simulink model "SG_GFOL_2020a"  (R2024a)
settings: Solver=ode1  StartTime=0.0  StopTime=Tsim  FixedStep=Ts  MaxStep=1e-4  RelTol=1e-4  EnableMultiTasking=on
values from neighbouring files (symbols this model uses):
  f1 = 50    [VSC_GF_SG_params.m]
  H = 5    [VSC_GF_SG_params.m]
  Inom_n2 = Sn_n2/Un_n2/sqrt(3)    [VSC_GF_SG_params.m]
  k_droop_f_n2 = 1/0.05    (= 20)    [VSC_GF_SG_params.m]
  ki_p_n2 = 1/tau_p    (= 5)    [VSC_GF_SG_params.m]
  ki_pll1 = kp_pll1/tau_pll_n1    [VSC_GF_SG_params.m]
  ki_pll_n2 = kp_pll_n2/tau_pll_n2    [VSC_GF_SG_params.m]
  ki_q_n2 = 1/tau_q    (= 5)    [VSC_GF_SG_params.m]
  ki_s_n2 = Rc_n2/taus_n2    (= 2048)    [VSC_GF_SG_params.m]
  kp_p_n2 = taus_n2/tau_p    (= 0.005)    [VSC_GF_SG_params.m]
  kp_pll1 = xi_pll_n1*2*omega_pll_n1/Vpeak    [VSC_GF_SG_params.m]
  kp_pll_n2 = xi_pll_n2*2*omega_pll_n2/Vpeak_n2    [VSC_GF_SG_params.m]
  kp_q_n2 = taus_n2/tau_q    (= 0.005)    [VSC_GF_SG_params.m]
  kp_s_n2 = Lc_n2/taus_n2    (= 130.379729381)    [VSC_GF_SG_params.m]
  Lac = Lpu*l*(Un1/Vl)^2    (= 0.105785123967)    [VSC_GF_SG_params.m]
  Lc_n2 = 0.2*Ln_n2    (= 0.130379729381)    [VSC_GF_SG_params.m]
  magnitud_delay = Ts    (= 5e-05)    [VSC_GF_SG_params.m]
  Pload_fnl = 400e6    (= 400000000)    [VSC_GF_SG_params.m]
  plots_step = Ts    (= 5e-05)    [VSC_GF_SG_params.m]
  Psg0_pu = Psg0/Pn    (= 0.4)    [VSC_GF_SG_params.m]
  Pvsc0 = Pload0 -Psg0    (= 200000000)    [VSC_GF_SG_params.m]
  Q_ref_n2 = 0e6    (= 0)    [VSC_GF_SG_params.m]
  Rac = Rpu*l*(Un1/Vl)^2    (= 3.17355371901)    [VSC_GF_SG_params.m]
  Rc_n2 = 0.01*Xn_n2    (= 2.048)    [VSC_GF_SG_params.m]
  Sn_n2 = Sn1    (= 500000000)    [VSC_GF_SG_params.m]
  Ssg = 500e6    (= 500000000)    [VSC_GF_SG_params.m]
  T_stp = 20    [VSC_GF_SG_params.m]
  tau_droop_fpll = 0.1    [VSC_GF_SG_params.m]
  tau_u = 40e-3    (= 0.04)    [VSC_GF_SG_params.m]
  Ts = 5e-5    (= 5e-05)    [VSC_GF_SG_params.m]
  Tsim = 40    [VSC_GF_SG_params.m]
  Un1 = 320e3    (= 320000)    [VSC_GF_SG_params.m]
  Vdcref_n1 = 640e3    (= 640000)    [VSC_GF_SG_params.m]
  Vpeak = Un1*sqrt(2/3)    [VSC_GF_SG_params.m]
  Vpeak_n1 = Un_n1/sqrt(3)*sqrt(2)    [VSC_GF_SG_params.m]
  Vpeak_n2 = Un_n2/sqrt(3)*sqrt(2)    [VSC_GF_SG_params.m]
  w_g1 = 2*pi*f1    (= 314.159265359)    [VSC_GF_SG_params.m]
  w_n2 = 2*pi*f_n2    (= 314.159265359)    [VSC_GF_SG_params.m]
undefined symbols (not defined in the file or in its folder): D11, Delta, k, magnitude, P_set, P_step, Pload_init, Q_set, Q_step, t_ramp, t_step_P, t_step_Q, tau_ramp, tau_wf
libraries: simulink x6, simulink_extras x6, spsSeriesRLCBranchLib x6, spsThreePhaseParallelRLCLoadLib x4, spsControlledVoltageSourceLib x4, spsCurrentMeasurementLib x4, spsControlledCurrentSourceLib x3, spsVoltageMeasurementLib x3, spsLoadFlowBusLib x2, slpidlib x2, spsGroundLib x2, spsSampleandHoldLib x1
(part 1 of 2)
settings Model: ExtModeTrigDuration=100  Creator=Enric  LastModifiedBy=citcea
settings SolverCC: SolverJacobianMethodControl=FullPerturbation  AlgebraicLoopSolver=TrustRegion
settings DataIOCC: LimitDataPoints=on  SaveOutput=off  ReturnWorkspaceOutputs=off  StateSaveName=tmp_raccel_xout  SignalLoggingName=tmp_raccel_logsout
settings OptimizationCC: EfficientMapNaN2IntZero=off  LifeSpan=inf
settings DebuggingCC: UnconnectedInputMsg=warning  UnconnectedOutputMsg=warning  UnconnectedLineMsg=warning  AllowSymbolicDim=off  SFUnexpectedBacktrackingDiag=warning  SFNoUnconditionalDefaultTransitionDiag=warning  SFExecutionAtInitializationDiag=none  ArithmeticOperatorsInVariantConditions=warning
settings HardwareCC: TargetBitPerPointer=64  TargetBitPerSizeT=64  TargetBitPerPtrDiffT=64  TargetLongLongMode=on  TargetIntDivRoundTo=Zero  TargetEndianess=LittleEndian  TargetWordSize=64  TargetHWDeviceType=MATLAB Host  ProdEqTarget=off
settings ModelReferenceCC: EnableRefExpFcnMdlSchedulingChecks=on  PropagateSignalLabelsOutOfModel=off
settings SFSimCC: SimUseLocalCustomCode=off  CustomCodeUndefinedFunction=UseInterfaceOnly
settings RTWCC: SystemTargetFile=raccel.tlc  TemplateMakefile=raccel_default_tmf  RTWVerbose=off  RTWUseLocalCustomCode=off  RTWUseSimCustomCode=on  GPUComputeCapability=3.5
settings CodeAppCC: GenerateComments=off  MaxIdLength=128  MangleLength=10  SimulinkBlockComments=off
settings RaccelTargetCC: InstructionSetFMA=off  OptimizeReductions=off  LogToMDFFile=off  ENABLE_SLEXEC_SSBRIDGE=0  RTWCAPISignals=off  RTWCAPIParams=on  RTWCAPIRootIO=off
settings ConfigComp: CovMetricSettings=dw  CovSaveCumulativeToWorkspaceVar=on  CovSaveSingleToWorkspaceVar=on  CovExternalEMLEnable=off
settings SimscapeCC: SimscapeNormalizeSystem=off

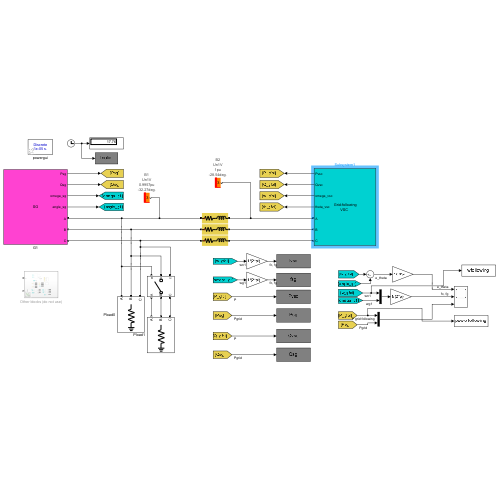
[thumbnail: Simulink's stored preview of the top-level diagram]
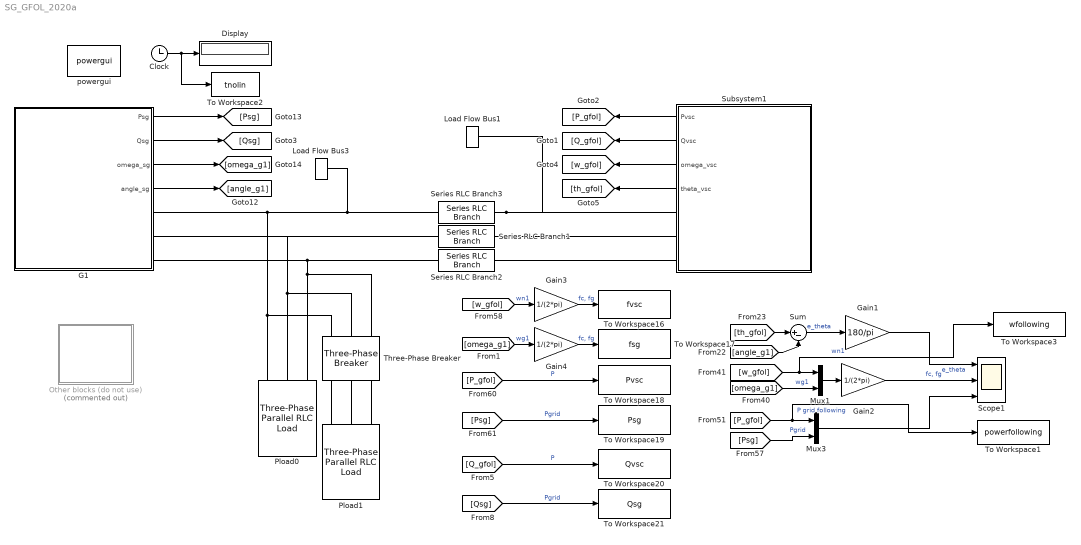
== system SG_GFOL_2020a ==
  Clock : Clock
  Display : Display
  G1 : Subsystem
      mask Display:
      | disp('SG')
      | %x = [0:0.001:1];
      | %y = 0.2*sin(10*x) + 0.5;
      | %plot(x,y)
  Gain1 : Gain  Gain=180/pi
  Gain2 : Gain  Gain=1/(2*pi)
  Gain3 : Gain  Gain=1/(2*pi)
  Gain4 : Gain  Gain=1/(2*pi)
  Load Flow Bus1 : spsLoadFlowBusLib/Load Flow Bus  LConnTagsString=a  Phases=single  Connectors=on one side  ID=B2  Vbase=Un1  Vref=1  Vangle=0  VLF=1  VLFb=1  VLFc=1  angleLF=-28.54  angleLFb=0  angleLFc=0
  Load Flow Bus3 : spsLoadFlowBusLib/Load Flow Bus  LConnTagsString=a  Phases=single  Connectors=on one side  ID=B1  Vbase=Un1  Vref=1  Vangle=0  VLF=0.9957  VLFb=1  VLFc=1  angleLF=-32.27  angleLFb=0  angleLFc=0
  Mux1 : Mux  Inputs=2
  Mux3 : Mux  Inputs=2
  Other blocks (do not use) : Subsystem  Commented=on
  Pload0 : spsThreePhaseParallelRLCLoadLib/Three-Phase Parallel RLC Load  LConnTagsString=A|B|C  Configuration=Y (grounded)  NominalVoltage=Vsg  Vabc=[1e3 1e3 1e3]  Vabcp=[1e3 1e3 1e3]  NominalFrequency=50  UnbalancedPower=off  ActivePower=Pload0  InductivePower=0  CapacitivePower=0  Pabc=[10e3 9e3 11e3]  QLabc=[100 90 110]  QCabc=[100 90 110]  Pabcp=[10e3 9e3 11e3]  QLabcp=[100 90 110]  QCabcp=[100 90 110]  Measurements=None  LoadType=constant Z
  Pload1 : spsThreePhaseParallelRLCLoadLib/Three-Phase Parallel RLC Load  LConnTagsString=A|B|C  Configuration=Y (grounded)  NominalVoltage=Vsg  Vabc=[1e3 1e3 1e3]  Vabcp=[1e3 1e3 1e3]  NominalFrequency=50  UnbalancedPower=off  ActivePower=Pload1  InductivePower=0  CapacitivePower=0  Pabc=[10e3 9e3 11e3]  QLabc=[100 90 110]  QCabc=[100 90 110]  Pabcp=[10e3 9e3 11e3]  QLabcp=[100 90 110]  QCabcp=[100 90 110]  Measurements=None  LoadType=constant Z
  Scope1 : Scope  NumInputPorts=3
  Series RLC Branch1 : spsSeriesRLCBranchLib/Series RLC Branch  LConnTagsString=__new0  RConnTagsString=__new0  BranchType=RL  Resistance=Rac  Inductance=Lac  SetiL0=off  InitialCurrent=0  Capacitance=0  Setx0=off  InitialVoltage=0  Measurements=None
  Series RLC Branch2 : spsSeriesRLCBranchLib/Series RLC Branch  LConnTagsString=__new0  RConnTagsString=__new0  BranchType=RL  Resistance=Rac  Inductance=Lac  SetiL0=off  InitialCurrent=0  Capacitance=0  Setx0=off  InitialVoltage=0  Measurements=None
  Series RLC Branch3 : spsSeriesRLCBranchLib/Series RLC Branch  LConnTagsString=__new0  RConnTagsString=__new0  BranchType=RL  Resistance=Rac  Inductance=Lac  SetiL0=off  InitialCurrent=0  Capacitance=0  Setx0=off  InitialVoltage=0  Measurements=None
  Subsystem1 : Subsystem
      mask Display: disp('VSC \n Grid-following')
  Sum : Sum  Inputs=|+-
  Three-Phase Breaker : spsThreePhaseBreakerLib/Three-Phase Breaker  InitialState=open  SwitchA=on  SwitchB=on  SwitchC=on  SwitchTimes=[T_stp 1000]  External=off  BreakerResistance=0.0001  SnubberResistance=inf  SnubberCapacitance=inf  Measurements=None
  To Workspace1 : ToWorkspace  VariableName=powerfollowing  SaveFormat=Timeseries  SampleTime=-1
  To Workspace16 : ToWorkspace  VariableName=fvsc  SampleTime=plots_step
  To Workspace17 : ToWorkspace  VariableName=fsg  SampleTime=plots_step
  To Workspace18 : ToWorkspace  VariableName=Pvsc  SampleTime=plots_step
  To Workspace19 : ToWorkspace  VariableName=Psg  SampleTime=plots_step
  To Workspace2 : ToWorkspace  VariableName=tnolin  SampleTime=plots_step
  To Workspace20 : ToWorkspace  VariableName=Qvsc  SampleTime=plots_step
  To Workspace21 : ToWorkspace  VariableName=Qsg  SampleTime=plots_step
  To Workspace3 : ToWorkspace  VariableName=wfollowing  SaveFormat=Timeseries  SampleTime=-1
  powergui : sps_lib/powergui  Priority=1  SimulationMode=Discrete  SampleTime=Ts  frequency=50  Iterations=50  frequencyindice=0  Pbase=100e6  ErrMax=0.0001  UnitsV=kV  UnitsW=MW  buscounter=0  FunctionMessages=off  echomessages=off  EnableUseOfTLC=off  CurrentSourceSwitches=off  DisableSnubberDevices=off  DisableRonSwitches=off  DisableVfSwitches=off  DisplayEquations=off  AutomaticDiscreteSolvers=off  SolverType=Tustin  Interpol=off  ExternalGateDelay=off  methode=off  Ts=0  x0status=blocks  SPID=off  SwTol=0  HookPort=off  NonlinearTolerance=1e-4  nMaxIteration=100  ContinueOnMaxIteration=off  RestoreLinks=warning  ResistiveCurrentMeasurement=off  Frange=[0:2:500]  Ylog=off  Xlog=on  ShowGrid=off  save=off  variable=ZData  structure=Vk  ZoomFFT=off  StartTime=2.01  cycles=3  DisplayStyle=1  fundamental=50  FreqAxis=off  MaxFrequency=1000  frequencyindicesteady=1  RmsSteady=1  display=off
  wires:
  Clock/1 -> To Workspace2/1, Display/1
  [th_gfol] -> Sum/1
  [angle_g1] -> Sum/2
  Sum/1 -> Gain1/1  "e_theta"
  [w_gfol] -> To Workspace3/1, Mux1/1  "wn1"
  [omega_g1] -> Mux1/2  "wg1"
  Mux1/1 -> Gain2/1
  Gain2/1 -> Scope1/2  "fc, fg"
  Gain1/1 -> Scope1/1  "e_theta"
  [P_gfol] -> To Workspace1/1, Mux3/1  "P grid following"
  [Psg] -> Mux3/2  "Pgrid"
  Mux3/1 -> Scope1/3
  [w_gfol] -> Gain3/1  "wn1"
  Gain3/1 -> To Workspace16/1  "fc, fg"
  Gain4/1 -> To Workspace17/1  "fc, fg"
  [omega_g1] -> Gain4/1  "wg1"
  [P_gfol] -> To Workspace18/1  "P"
  [Psg] -> To Workspace19/1  "Pgrid"
  G1/1(Psg) -> [Psg]
  G1/3(omega_sg) -> [omega_g1]
  G1/4(angle_sg) -> [angle_g1]
  Subsystem1/4(theta_vsc) -> [th_gfol]
  Subsystem1/3(omega_vsc) -> [w_gfol]
  Subsystem1/1(Pvsc) -> [P_gfol]
  Subsystem1/2(Qvsc) -> [Q_gfol]
  [Qsg] -> To Workspace21/1  "Pgrid"
  [Q_gfol] -> To Workspace20/1  "P"
  G1/2(Qsg) -> [Qsg]
  connections:
  Series RLC Branch1/LConn1 -- G1/RConn2 -- Three-Phase Breaker/RConn2 -- Pload0/LConn2
  Series RLC Branch3/RConn1 -- Subsystem1/RConn1 -- Load Flow Bus1/LConn1
  Subsystem1/RConn2 -- Series RLC Branch1/RConn1
  Subsystem1/RConn3 -- Series RLC Branch2/RConn1
  Load Flow Bus3/LConn1 -- Series RLC Branch3/LConn1 -- Three-Phase Breaker/RConn1 -- Pload0/LConn1 -- G1/RConn1
  Three-Phase Breaker/LConn1 -- Pload1/LConn1
  Pload1/LConn2 -- Three-Phase Breaker/LConn2
  Three-Phase Breaker/LConn3 -- Pload1/LConn3
  Series RLC Branch2/LConn1 -- Three-Phase Breaker/RConn3 -- Pload0/LConn3 -- G1/RConn3

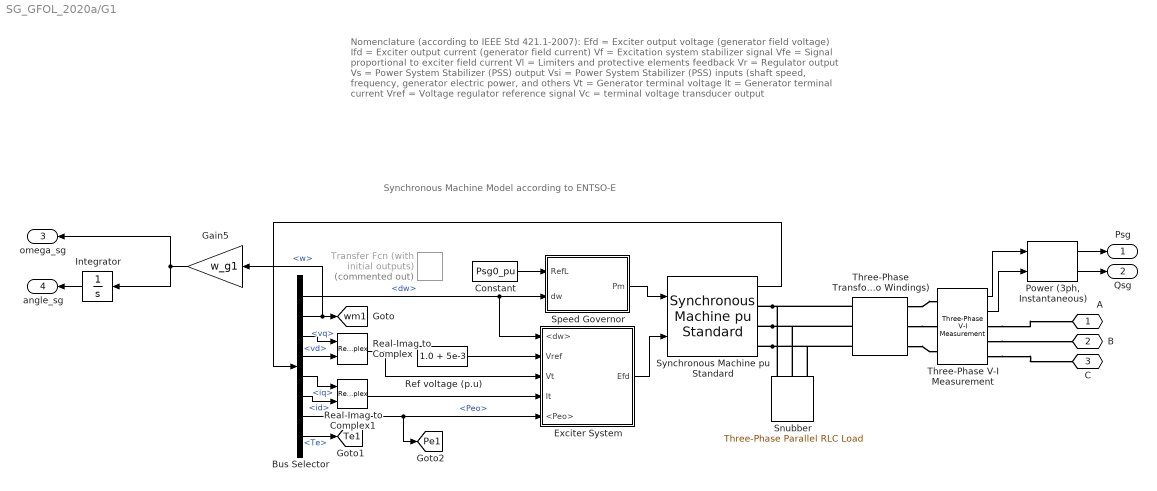
== system SG_GFOL_2020a/G1 ==
  note: Synchronous Machine Model according to ENTSO-E
  note: Nomenclature (according to IEEE Std 421.1-2007):
      | Efd = Exciter output voltage (generator field voltage)
      | Ifd = Exciter output current (generator field current)
      | Vf = Excitation system stabilizer signal
      | Vfe = Signal proportional to exciter field current
      | Vl = Limiters and protective elements feedback
      | Vr = Regulator output
      | Vs = Power System Stabilizer (PSS) output
      | Vsi = Power System Stabilizer (PSS) inputs (shaft speed, frequency, generator electric power, and others
      | Vt = Generator terminal voltage
      | It = Generator terminal current
      | Vref = Voltage regulator reference signal
      | Vc = terminal voltage transducer output
  Bus Selector : BusSelector  OutputSignals=dw,w,vq,vd,iq,id,Peo,Te
  Constant : Constant  Value=Psg0_pu
  Exciter System : Subsystem
  Gain5 : Gain  Gain=w_g1
  Integrator : Integrator
  "Power (3ph, Instantaneous)" : spsPower3phInstantaneousLib/Power (3ph, Instantaneous)
  Real-Imag to Complex : RealImagToComplex
  Real-Imag to Complex1 : RealImagToComplex
  Ref voltage (p.u) : Constant  Value=1.0 + 5e-3
  Snubber : spsThreePhaseParallelRLCLoadLib/Three-Phase Parallel RLC Load  LConnTagsString=A|B|C  Configuration=Y (grounded)  NominalVoltage=Un1  Vabc=[1e3 1e3 1e3]  Vabcp=[1e3 1e3 1e3]  NominalFrequency=f1  UnbalancedPower=off  ActivePower=Ssg*0.01  InductivePower=0  CapacitivePower=0  Pabc=[10e3 9e3 11e3]  QLabc=[100 90 110]  QCabc=[100 90 110]  Pabcp=[10e3 9e3 11e3]  QLabcp=[100 90 110]  QCabcp=[100 90 110]  Measurements=None  LoadType=constant Z
  Speed Governor : Subsystem  mask{R=0.05, T1=0.5, T2=3, T3=10, Dt=0, Vmin=0, Vmax=10, P0=Psg0_pu}
      mask prompts: R "Controller droop (R)"; T1 "Governor time constant (T1)(sec)"; T2 "Turbine derivative time constant (T2)(sec)"; T3 "Turbine delay time constant (T3)(sec)"; Dt "Frictional losses factor (Dt)"; Vmin "Minimum gate limit (Vmin)(p.u)"; Vmax "Maximum gate limit (Vmax)(p.u)"; P0 "Initial power (p.u)"
      mask Display:
      | disp('TGOV')
      | 
      | port_label('input',1,'Pref')
      | port_label('input',2,'dw')
      | 
      | port_label('output',1,'Pm')
  Synchronous Machine pu Standard : spsSynchronousMachinepuStandardLib/Synchronous Machine pu Standard  PresetModel=No  MechanicalLoad=Mechanical power Pm  ShowDetailedParameters=on  RotorType=Salient-pole  Units=per unit standard parameters  MeasurementBus=on  NominalParameters=[Ssg Un1 f1]  Reactances1=[ 1.81, 0.3, 0.23, 1.76, 0.65, 0.25, 0.15 ]  Reactances2=[1.25 0.333 0.292 1.0 0.292 0.15]  dAxisTimeConstants=Open-circuit  qAxisTimeConstants=Open-circuit  TimeConstants1="[5  0.002  0.002]"  TimeConstants2=[ 8.0, 0.03, 1.0, 0.07 ]  TimeConstants3="[  4.49  0.0681  0.0513  ]"  TimeConstants4=[ 8.0, 0.03, 0.3371, 0.0295 ]  TimeConstants5=[ 1.01, 0.053, 0.1 ]  TimeConstants6=[ 1.3201, 0.023, 1.0, 0.07 ]  TimeConstants7=[0.012 0.003 0.003]  TimeConstants8=[ 1.3201, 0.0231, 0.3371, 0.0295 ]  StatorResistance=0.01  Mechanical=[H 0 2]  PolePairs=20  InitialConditions=[0 -68.7735 0.408291 0.408291 0.408291 -5.73726 -125.737 114.263 1.16721]  SetSaturation=off  Saturation=[0.6404,0.7127,0.8441,0.9214,0.9956,1.082,1.19,1.316,1.457;0.7,0.7698,0.8872,0.9466,0.9969,1.046,1.1,1.151,1.201]  LoadFlowParameters=[1,0,0,0,0]  TsPowergui=0  TsBlock=-1  IterativeModel=Trapezoidal non iterative  IterativeDiscreteModel=Trapezoidal non iterative  BusType=swing  Pref=0  Qref=0  Qmin=-inf  Qmax=inf  PLF=0  QLF=0
  Three-Phase Transformer (Two Windings) : spsThreePhaseTransformerTwoWindingsLib/Three-Phase Transformer (Two Windings)  Winding1Connection=Delta (D11)  Winding2Connection=Yg  CoreType=Three single-phase transformers  SetSaturation=off  Hysteresis=off  DataFile='hysteresis'  SetInitialFlux=off  Measurements=None  UNITS=pu  NominalPower=[Ssg , f1 ]  Winding1=[Un1 0.00125 0.05]  Winding2=[Un1 0.00125 0.05]  Rm=5000  Lm=5000  L0=0.5  Saturation=[ 0,0 ; 0.0024,1.2 ; 1.0,1.52 ]  InitialFluxes=[ 0.8 , -0.8 , 0.7 ]  BreakLoop=off  DiscreteSolver=Trapezoidal iterative  DataType=off  TransfoNumber=1
  Three-Phase V-I Measurement : spsThreePhaseVIMeasurementLib/Three-Phase V-I Measurement  VoltageMeasurement=phase-to-ground  SetLabelV=off  LabelV=Vabc  Vpu=off  VpuLL=off  CurrentMeasurement=yes  SetLabelI=off  LabelI=Iabc  Ipu=off  Pbase=100e6  Vbase=500e3  OutputType=Complex  PhasorSimulation=off  PSBequivalent=0
  Transfer Fcn (with initial outputs) : simulink_extras/Additional Linear/Transfer Fcn (with initial outputs)  Commented=on  N=[-1.8]  D="[1  0]"  Y0=0.0705  U0=0
  A : PMIOPort  Side=Right
  B : PMIOPort  Port=2  Side=Right
  C : PMIOPort  Port=3  Side=Right
  Psg : Outport
  Qsg : Outport  Port=2
  omega_sg : Outport  Port=3
  angle_sg : Outport  Port=4
  tag scope: Pe1=global, Te1=global, wm1=global
  wires:
  Ref voltage (p.u)/1 -> Exciter System/2(Vref)
  Bus Selector/1 -> Exciter System/1(<dw>), Speed Governor/2(dw)  "<dw>"
  Bus Selector/4 -> Real-Imag to Complex/2  "<vd>"
  Bus Selector/3 -> Real-Imag to Complex/1  "<vq>"
  Bus Selector/5 -> Real-Imag to Complex1/1  "<iq>"
  Bus Selector/6 -> Real-Imag to Complex1/2  "<id>"
  Real-Imag to Complex/1 -> Exciter System/3(Vt)
  Real-Imag to Complex1/1 -> Exciter System/4(It)
  Bus Selector/7 -> Exciter System/5(<Peo>), [Pe1]  "<Peo>"
  Bus Selector/8 -> [Te1]  "<Te>"
  Speed Governor/1(Pm) -> Synchronous Machine pu Standard/1
  Exciter System/1(Efd) -> Synchronous Machine pu Standard/2
  Synchronous Machine pu Standard/1 -> Bus Selector/1
  Constant/1 -> Speed Governor/1(RefL)
  Bus Selector/2 -> Gain5/1, [wm1]  "<w>"
  Integrator/1 -> angle_sg/1
  Gain5/1 -> Integrator/1, omega_sg/1
  Three-Phase V-I Measurement/2 -> "Power (3ph, Instantaneous)"/2
  Three-Phase V-I Measurement/1 -> "Power (3ph, Instantaneous)"/1
  "Power (3ph, Instantaneous)"/1 -> Psg/1
  "Power (3ph, Instantaneous)"/2 -> Qsg/1
  connections:
  Synchronous Machine pu Standard/RConn1 -- Three-Phase Transformer (Two Windings)/LConn1 -- Snubber/LConn1
  Synchronous Machine pu Standard/RConn3 -- Three-Phase Transformer (Two Windings)/LConn3 -- Snubber/LConn3
  Synchronous Machine pu Standard/RConn2 -- Three-Phase Transformer (Two Windings)/LConn2 -- Snubber/LConn2
  Three-Phase Transformer (Two Windings)/RConn2 -- Three-Phase V-I Measurement/LConn2
  Three-Phase Transformer (Two Windings)/RConn1 -- Three-Phase V-I Measurement/LConn1
  Three-Phase Transformer (Two Windings)/RConn3 -- Three-Phase V-I Measurement/LConn3
  Three-Phase V-I Measurement/RConn1 -- A/RConn1
  Three-Phase V-I Measurement/RConn2 -- B/RConn1
  Three-Phase V-I Measurement/RConn3 -- C/RConn1

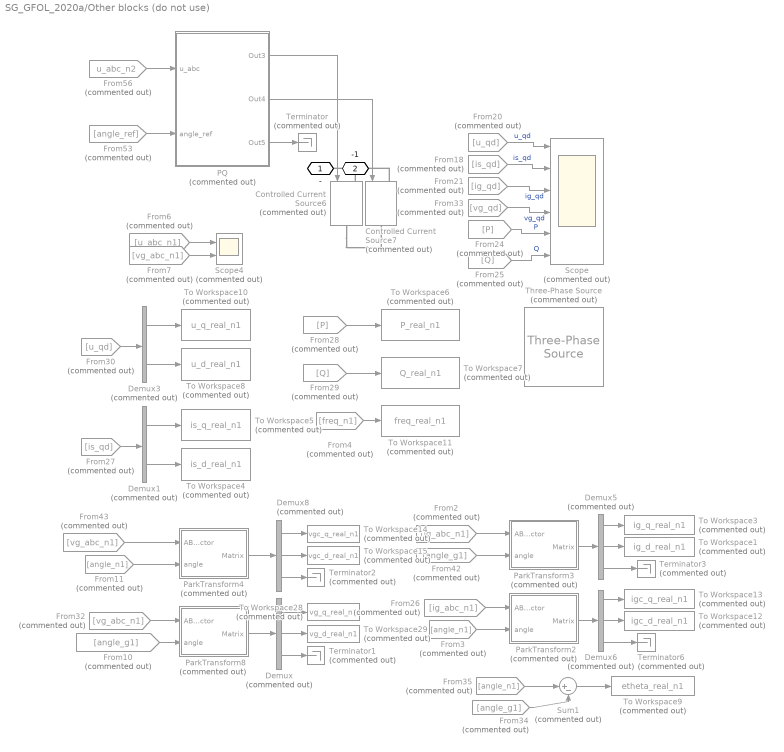
== system SG_GFOL_2020a/Other blocks (do not use) ==
  Controlled Current Source6 : spsControlledCurrentSourceLib/Controlled Current Source  Commented=on  Initialize=off  Source_Type=AC  Amplitude=0  Phase=0  Frequency=0  Measurements=None
  Controlled Current Source7 : spsControlledCurrentSourceLib/Controlled Current Source  Commented=on  Initialize=off  Source_Type=AC  Amplitude=0  Phase=0  Frequency=0  Measurements=None
  Demux{,5..6,8} (4 alike) : Demux  Commented=on  Outputs=3
  Demux1 : Demux  Commented=on  Outputs=2
  Demux3 : Demux  Commented=on  Outputs=2
  From10 : From  Commented=on  GotoTag=angle_g1
  From11 : From  Commented=on  GotoTag=angle_n1
  From18 : From  Commented=on  GotoTag=is_qd
  From2 : From  Commented=on  GotoTag=ig_abc_n1
  From20 : From  Commented=on  GotoTag=u_qd
  From21 : From  Commented=on  GotoTag=ig_qd
  From24 : From  Commented=on  GotoTag=P
  From25 : From  Commented=on  GotoTag=Q
  From26 : From  Commented=on  GotoTag=ig_abc_n1
  From27 : From  Commented=on  GotoTag=is_qd
  From28 : From  Commented=on  GotoTag=P
  From29 : From  Commented=on  GotoTag=Q
  From3 : From  Commented=on  GotoTag=angle_n1
  From30 : From  Commented=on  GotoTag=u_qd
  From32 : From  Commented=on  GotoTag=vg_abc_n1
  From33 : From  Commented=on  GotoTag=vg_qd
  From34 : From  Commented=on  GotoTag=angle_g1
  From35 : From  Commented=on  GotoTag=angle_n1
  From4 : From  Commented=on  GotoTag=freq_n1
  From42 : From  Commented=on  GotoTag=angle_g1
  From43 : From  Commented=on  GotoTag=vg_abc_n1
  From53 : From  Commented=on  GotoTag=angle_ref
  From56 : From  Commented=on  GotoTag=u_abc_n2  TagVisibility=global
  From6 : From  Commented=on  GotoTag=u_abc_n1
  From7 : From  Commented=on  GotoTag=vg_abc_n1
  PQ : Subsystem  Commented=on
  ParkTransform2 : Subsystem  Commented=on  mask(Gerard){}
      mask help:
      | This block applies the park transfomation from a desired vector.
      | The input Xabc refers to the vector in the ABC frame, and the second input is the angle used in the transformation.
      | The output is the vector in the qd0 frame.
      mask Display:
      | port_label('output',1,'Xqd0')
      | port_label('input',1,'Xabc')
      | port_label('input',2,'angle')
  ParkTransform3 : Subsystem  Commented=on  mask(Gerard){}
      mask help:
      | This block applies the park transfomation from a desired vector.
      | The input Xabc refers to the vector in the ABC frame, and the second input is the angle used in the transformation.
      | The output is the vector in the qd0 frame.
      mask Display:
      | port_label('output',1,'Xqd0')
      | port_label('input',1,'Xabc')
      | port_label('input',2,'angle')
  ParkTransform4 : Subsystem  Commented=on  mask(Gerard){}
      mask help:
      | This block applies the park transfomation from a desired vector.
      | The input Xabc refers to the vector in the ABC frame, and the second input is the angle used in the transformation.
      | The output is the vector in the qd0 frame.
      mask Display:
      | port_label('output',1,'Xqd0')
      | port_label('input',1,'Xabc')
      | port_label('input',2,'angle')
  ParkTransform8 : Subsystem  Commented=on  mask(Gerard){}
      mask help:
      | This block applies the park transfomation from a desired vector.
      | The input Xabc refers to the vector in the ABC frame, and the second input is the angle used in the transformation.
      | The output is the vector in the qd0 frame.
      mask Display:
      | port_label('output',1,'Xqd0')
      | port_label('input',1,'Xabc')
      | port_label('input',2,'angle')
  Scope : Scope  Commented=on  NumInputPorts=6
  Scope4 : Scope  Commented=on  NumInputPorts=2
  Sum1 : Sum  Commented=on  Inputs=|+-
  Terminator{,1..3,6} (5 alike) : Terminator  Commented=on
  Three-Phase Source : spsThreePhaseSourceLib/Three-Phase Source  Commented=on  InternalConnection=Yg  VoltagePhases=off  Voltage=(320000)*1  PhaseAngle=-28.5377  Voltage_phases=[25e3 25e3 25e3]/sqrt(3)  PhaseAngles_phases=[0 -120 +120]  Frequency=f1  NonIdealSource=on  SpecifyImpedance=off  Resistance=0  Inductance=0  ShortCircuitLevel=100e6  BaseVoltage=Un1  XRratio=7  BusType=PV  Pref=Pvsc0  Qref=0  Prefabc=[10e3, 10e3, 10e3]  Qrefabc=[0, 0, 0]  Qmin=-inf  Qmax=inf
  To Workspace1 : ToWorkspace  Commented=on  VariableName=ig_d_real_n1  SampleTime=plots_step
  To Workspace10 : ToWorkspace  Commented=on  VariableName=u_q_real_n1  SampleTime=plots_step
  To Workspace11 : ToWorkspace  Commented=on  VariableName=freq_real_n1  SampleTime=plots_step
  To Workspace12 : ToWorkspace  Commented=on  VariableName=igc_d_real_n1  SampleTime=plots_step
  To Workspace13 : ToWorkspace  Commented=on  VariableName=igc_q_real_n1  SampleTime=plots_step
  To Workspace14 : ToWorkspace  Commented=on  VariableName=vgc_q_real_n1  SampleTime=plots_step
  To Workspace15 : ToWorkspace  Commented=on  VariableName=vgc_d_real_n1  SampleTime=plots_step
  To Workspace28 : ToWorkspace  Commented=on  VariableName=vg_q_real_n1  SampleTime=plots_step
  To Workspace29 : ToWorkspace  Commented=on  VariableName=vg_d_real_n1  SampleTime=plots_step
  To Workspace3 : ToWorkspace  Commented=on  VariableName=ig_q_real_n1  SampleTime=plots_step
  To Workspace4 : ToWorkspace  Commented=on  VariableName=is_d_real_n1  SampleTime=plots_step
  To Workspace5 : ToWorkspace  Commented=on  VariableName=is_q_real_n1  SampleTime=plots_step
  To Workspace6 : ToWorkspace  Commented=on  VariableName=P_real_n1  SampleTime=plots_step
  To Workspace7 : ToWorkspace  Commented=on  VariableName=Q_real_n1  SampleTime=plots_step
  To Workspace8 : ToWorkspace  Commented=on  VariableName=u_d_real_n1  SampleTime=plots_step
  To Workspace9 : ToWorkspace  Commented=on  VariableName=etheta_real_n1  SampleTime=plots_step
  - : PMIOPort  Side=Left
  -1 : PMIOPort  Port=2  Side=Left
  wires:
  Demux8/2 -> To Workspace15/1
  From7/1 -> Scope4/2
  Demux6/2 -> To Workspace12/1
  From4/1 -> To Workspace11/1
  ParkTransform8/1(Matrix) -> Demux/1
  From27/1 -> Demux1/1
  Demux5/1 -> To Workspace3/1
  From26/1 -> ParkTransform2/1(ABC vector)
  From56/1 -> PQ/1(u_abc)
  From10/1 -> ParkTransform8/2(angle)
  From42/1 -> ParkTransform3/2(angle)
  From11/1 -> ParkTransform4/2(angle)
  Demux5/2 -> To Workspace1/1
  Sum1/1 -> To Workspace9/1
  PQ/3(Out5) -> Terminator/1
  From3/1 -> ParkTransform2/2(angle)
  Demux/3 -> Terminator1/1
  PQ/2(Out4) -> Controlled Current Source7/1
  From33/1 -> Scope/4  "vg_qd"
  Demux1/2 -> To Workspace4/1
  From20/1 -> Scope/1  "u_qd"
  From34/1 -> Sum1/2
  From53/1 -> PQ/2(angle_ref)
  From28/1 -> To Workspace6/1
  Demux3/2 -> To Workspace8/1
  ParkTransform2/1(Matrix) -> Demux6/1
  Demux1/1 -> To Workspace5/1
  From2/1 -> ParkTransform3/1(ABC vector)
  From25/1 -> Scope/6  "Q"
  Demux/2 -> To Workspace29/1
  PQ/1(Out3) -> Controlled Current Source6/1
  From24/1 -> Scope/5  "P"
  ParkTransform3/1(Matrix) -> Demux5/1
  From35/1 -> Sum1/1
  Demux8/3 -> Terminator2/1
  From21/1 -> Scope/3  "ig_qd"
  Demux5/3 -> Terminator3/1
  Demux/1 -> To Workspace28/1
  From43/1 -> ParkTransform4/1(ABC vector)
  Demux3/1 -> To Workspace10/1
  From29/1 -> To Workspace7/1
  From30/1 -> Demux3/1
  From32/1 -> ParkTransform8/1(ABC vector)
  From6/1 -> Scope4/1
  Demux6/1 -> To Workspace13/1
  ParkTransform4/1(Matrix) -> Demux8/1
  Demux6/3 -> Terminator6/1
  Demux8/1 -> To Workspace14/1
  From18/1 -> Scope/2  "is_qd"
  connections:
  Controlled Current Source6/LConn1 -- -/RConn1
  Controlled Current Source6/RConn1 -- Controlled Current Source7/RConn1
  Controlled Current Source7/LConn1 -- -1/RConn1

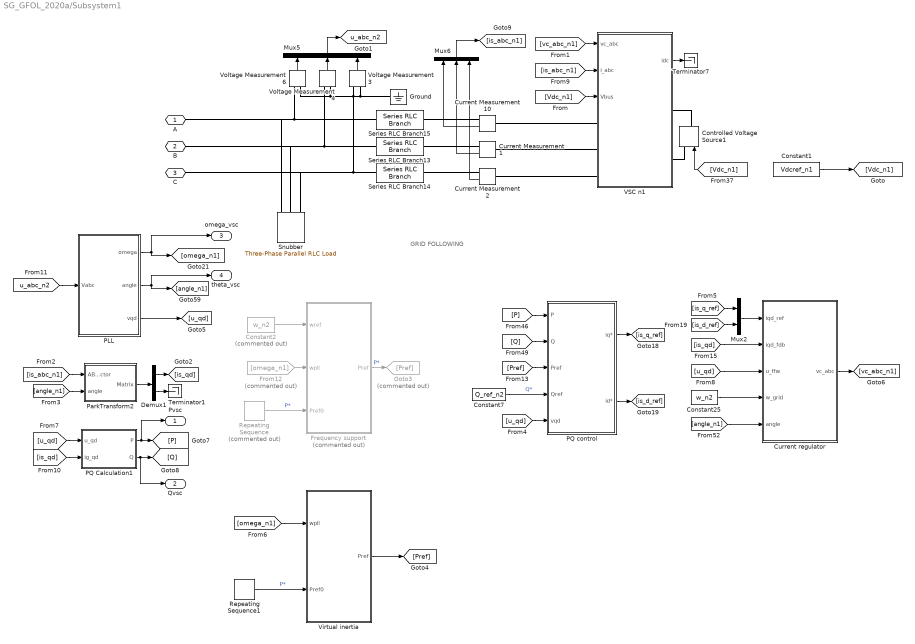
== system SG_GFOL_2020a/Subsystem1 ==
  note: GRID FOLLOWING
  Constant1 : Constant  Value=Vdcref_n1
  Constant2 : Constant  Commented=on  Value=w_n2
  Constant25 : Constant  Value=w_n2
  Constant7 : Constant  Value=Q_ref_n2
  Controlled Voltage Source1 : spsControlledVoltageSourceLib/Controlled Voltage Source  Initialize=on  Source_Type=DC  Amplitude=Vdcref_n1  Phase=0  Frequency=0  Measurements=None
  Current Measurement1 : spsCurrentMeasurementLib/Current Measurement  PhasorSimulation=off  OutputType=Complex  PSBequivalent=0
  Current Measurement10 : spsCurrentMeasurementLib/Current Measurement  PhasorSimulation=off  OutputType=Complex  PSBequivalent=0
  Current Measurement2 : spsCurrentMeasurementLib/Current Measurement  PhasorSimulation=off  OutputType=Complex  PSBequivalent=0
  Current regulator : Subsystem
  Demux1 : Demux  Outputs=2
  Frequency support : Subsystem  Commented=on
  From12 : From  Commented=on  GotoTag=omega_n1
  Goto3 : Goto  Commented=on  GotoTag=Pref
  Ground : spsGroundLib/Ground  LConnTagsString=a
  Mux2 : Mux  Inputs=2
  Mux5 : Mux  Inputs=3
  Mux6 : Mux  Inputs=3
  PLL : Subsystem
  PQ Calculation1 : Subsystem
  PQ control : Subsystem
  ParkTransform2 : Subsystem  mask(Gerard){}
      mask help:
      | This block applies the park transfomation from a desired vector.
      | The input Xabc refers to the vector in the ABC frame, and the second input is the angle used in the transformation.
      | The output is the vector in the qd0 frame.
      mask Display:
      | port_label('output',1,'Xqd0')
      | port_label('input',1,'Xabc')
      | port_label('input',2,'angle')
  Repeating Sequence : simulink/Sources/Repeating Sequence  Commented=on  rep_seq_t=[0 0.05 0.1 Tsim]  rep_seq_y=[0 0 Pvsc0 Pvsc0]
  Repeating Sequence1 : simulink/Sources/Repeating Sequence  rep_seq_t=[0 0.05 0.1 Tsim]  rep_seq_y=[0 0 Pvsc0 Pvsc0]
  Series RLC Branch13 : spsSeriesRLCBranchLib/Series RLC Branch  LConnTagsString=__new0  RConnTagsString=__new0  BranchType=RL  Resistance=Rc_n2  Inductance=Lc_n2  SetiL0=off  InitialCurrent=0  Capacitance=0  Setx0=off  InitialVoltage=0  Measurements=None
  Series RLC Branch14 : spsSeriesRLCBranchLib/Series RLC Branch  LConnTagsString=__new0  RConnTagsString=__new0  BranchType=RL  Resistance=Rc_n2  Inductance=Lc_n2  SetiL0=off  InitialCurrent=0  Capacitance=0  Setx0=off  InitialVoltage=0  Measurements=None
  Series RLC Branch15 : spsSeriesRLCBranchLib/Series RLC Branch  LConnTagsString=__new0  RConnTagsString=__new0  BranchType=RL  Resistance=Rc_n2  Inductance=Lc_n2  SetiL0=off  InitialCurrent=0  Capacitance=0  Setx0=off  InitialVoltage=0  Measurements=None
  Snubber : spsThreePhaseParallelRLCLoadLib/Three-Phase Parallel RLC Load  LConnTagsString=A|B|C  Configuration=Y (grounded)  NominalVoltage=Un1  Vabc=[1e3 1e3 1e3]  Vabcp=[1e3 1e3 1e3]  NominalFrequency=f1  UnbalancedPower=off  ActivePower=Sn_n2*0.01  InductivePower=0  CapacitivePower=0  Pabc=[10e3 9e3 11e3]  QLabc=[100 90 110]  QCabc=[100 90 110]  Pabcp=[10e3 9e3 11e3]  QLabcp=[100 90 110]  QCabcp=[100 90 110]  Measurements=None  LoadType=constant Z
  Terminator1 : Terminator
  Terminator7 : Terminator
  VSC n1 : Subsystem
  Virtual inertia : Subsystem
  Voltage Measurement3 : spsVoltageMeasurementLib/Voltage Measurement  PhasorSimulation=off  OutputType=Complex  PSBequivalent=0
  Voltage Measurement4 : spsVoltageMeasurementLib/Voltage Measurement  PhasorSimulation=off  OutputType=Complex  PSBequivalent=0
  Voltage Measurement6 : spsVoltageMeasurementLib/Voltage Measurement  PhasorSimulation=off  OutputType=Complex  PSBequivalent=0
  A : PMIOPort  Side=Right
  B : PMIOPort  Port=2  Side=Right
  C : PMIOPort  Port=3  Side=Right
  Pvsc : Outport
  Qvsc : Outport  Port=2
  omega_vsc : Outport  Port=3
  theta_vsc : Outport  Port=4
  tag scope: u_abc_n2=global
  wires:
  [is_abc_n1] -> ParkTransform2/1(ABC vector)
  Demux1/1 -> [is_qd]
  Demux1/2 -> Terminator1/1
  [is_qd] -> PQ Calculation1/2(ig_qd)
  PQ Calculation1/1(P) -> Pvsc/1, [P]
  [angle_n1] -> ParkTransform2/2(angle)
  PQ Calculation1/2(Q) -> Qvsc/1, [Q]
  [u_qd] -> PQ Calculation1/1(u_qd)
  ParkTransform2/1(Matrix) -> Demux1/1
  [is_qd] -> Current regulator/2(iqd_fdb)
  [angle_n1] -> Current regulator/5(angle)
  PQ control/2(id*) -> [is_d_ref]
  Mux2/1 -> Current regulator/1(iqd_ref)
  Current regulator/1(vc_abc) -> [vc_abc_n1]
  PQ control/1(iq*) -> [is_q_ref]
  Constant25/1 -> Current regulator/4(w_grid)
  [u_qd] -> Current regulator/3(u_ffw)
  [is_d_ref] -> Mux2/2
  [is_q_ref] -> Mux2/1
  Voltage Measurement3/1 -> Mux5/3
  Voltage Measurement4/1 -> Mux5/2
  Current Measurement2/1 -> Mux6/3
  VSC n1/1(idc) -> Terminator7/1
  Constant1/1 -> [Vdc_n1]
  Current Measurement1/1 -> Mux6/2
  [Vdc_n1] -> Controlled Voltage Source1/1
  Current Measurement10/1 -> Mux6/1
  Mux6/1 -> [is_abc_n1]
  Voltage Measurement6/1 -> Mux5/1
  [Vdc_n1] -> VSC n1/3(Vbus)
  [vc_abc_n1] -> VSC n1/1(vc_abc)
  Mux5/1 -> [u_abc_n2]
  [is_abc_n1] -> VSC n1/2(i_abc)
  [P] -> PQ control/1(P)
  [Q] -> PQ control/2(Q)
  Constant7/1 -> PQ control/4(Qref)  "Q*"
  [u_abc_n2] -> PLL/1(Vabc)
  PLL/2(angle) -> [angle_n1], theta_vsc/1
  PLL/1(omega) -> [omega_n1], omega_vsc/1
  PLL/3(vqd) -> [u_qd]
  [u_qd] -> PQ control/5(vqd)
  Repeating Sequence/1 -> Frequency support/3(Pref0)  "P*"
  Frequency support/1(Pref) -> Goto3/1  "P*"
  [Pref] -> PQ control/3(Pref)
  From12/1 -> Frequency support/2(wpll)
  Constant2/1 -> Frequency support/1(wref)
  Virtual inertia/1(Pref) -> [Pref]
  [omega_n1] -> Virtual inertia/1(wpll)
  Repeating Sequence1/1 -> Virtual inertia/2(Pref0)  "P*"
  connections:
  VSC n1/RConn2 -- Controlled Voltage Source1/LConn1
  Current Measurement2/RConn1 -- Series RLC Branch14/RConn1
  Voltage Measurement3/LConn2 -- Voltage Measurement6/LConn2 -- Voltage Measurement4/LConn2 -- Ground/LConn1
  Controlled Voltage Source1/RConn1 -- VSC n1/RConn1
  VSC n1/LConn1 -- Current Measurement10/LConn1
  Current Measurement2/LConn1 -- VSC n1/LConn3
  Voltage Measurement3/LConn1 -- Snubber/LConn3 -- C/RConn1 -- Series RLC Branch14/LConn1
  Current Measurement1/LConn1 -- VSC n1/LConn2
  Current Measurement10/RConn1 -- Series RLC Branch15/RConn1
  Series RLC Branch15/LConn1 -- A/RConn1 -- Snubber/LConn1 -- Voltage Measurement6/LConn1
  Current Measurement1/RConn1 -- Series RLC Branch13/RConn1
  Series RLC Branch13/LConn1 -- B/RConn1 -- Snubber/LConn2 -- Voltage Measurement4/LConn1

== system SG_GFOL_2020a/G1/Exciter System ==
  <dw> : Inport
  Vref : Inport  Port=2
  Vt : Inport  Port=3
  It : Inport  Port=4
  <Peo> : Inport  Port=5
  PSS1 : Subsystem  mask{Ks1=20, Ks2=0.1564, Ks3=1, Tw1=2, Tw2=2, Tw3=2, Tw4=0, T1=0.25, T2=0.2, T3=0.15, T4=0.1, T6=0, T7=2, T8=0.5, T9=0.1, Vstmin=-0.10, Vstmax=0.10, N=0, M=0, IC1=1, IC2=3}
      mask prompts: Ks1 "PSS gain (Ks1)"; Ks2 "2nd signal transducer factor(Ks2)"; Ks3 "washouts coupling factor (Ks3)"; Tw1 "1st washout 1th time constant (Tw1)(sec)"; Tw2 "1st washout 2nd time constant (Tw2)(sec)"; Tw3 "2nd washout 1st time constant (Tw3)(sec)"; Tw4 "2nd washout 2nd time constant (Tw4)(sec)"; T1 "1st lead-lag derivative time constant (T1)(sec)"; T2 "1st lead-lag delay time constant(T2)(sec)"; T3 "2nd lead-lag derivative time constant(T3)(sec)"; T4 "2nd lead-lag delay time constant(T4)(sec)"; T6 "1st signal transducer time constant(T6)(sec)"; T7 "2nd signal transducer time constant(T7)(sec)"; T8 "ramp tracking filter deriv. time constant(T8)(sec)"; T9 "ramp tracking filter delay time constant(T9)(sec)"; Vstmin "controller minimum output(Vstmin)"; Vstmax "controller maximum output(Vstmax)"; N "ramp tracking filter (N)"; M "ramp tracking filter (M)"; IC1 "1st input selector (IC1)"; IC2 "2nd input selector (IC2)"
      mask Display:
      | disp('PSS2A')
      | 
      | port_label('input',1,'dw')
      | port_label('input',2,'Pg')
      | %port_label('input',3,'Vs')
      | 
      | port_label('output',1,'Vs')
  PSS1 backup : Subsystem  Commented=on  mask{Ks1=10, Ks2=0.1564, Ks3=1, Tw1=2, Tw2=2, Tw3=2, Tw4=0, T1=0.25, T2=0.03, T3=0.15, T4=0.015, T6=0, T7=2, T8=0.5, T9=0.1, Vstmin=-0.1, Vstmax=0.1, N=0, M=0, IC1=1, IC2=3}
      mask prompts: Ks1 "PSS gain (Ks1)"; Ks2 "2nd signal transducer factor(Ks2)"; Ks3 "washouts coupling factor (Ks3)"; Tw1 "1st washout 1th time constant (Tw1)(sec)"; Tw2 "1st washout 2nd time constant (Tw2)(sec)"; Tw3 "2nd washout 1st time constant (Tw3)(sec)"; Tw4 "2nd washout 2nd time constant (Tw4)(sec)"; T1 "1st lead-lag derivative time constant (T1)(sec)"; T2 "1st lead-lag delay time constant(T2)(sec)"; T3 "2nd lead-lag derivative time constant(T3)(sec)"; T4 "2nd lead-lag delay time constant(T4)(sec)"; T6 "1st signal transducer time constant(T6)(sec)"; T7 "2nd signal transducer time constant(T7)(sec)"; T8 "ramp tracking filter deriv. time constant(T8)(sec)"; T9 "ramp tracking filter delay time constant(T9)(sec)"; Vstmin "controller minimum output(Vstmin)"; Vstmax "controller maximum output(Vstmax)"; N "ramp tracking filter (N)"; M "ramp tracking filter (M)"; IC1 "1st input selector (IC1)"; IC2 "2nd input selector (IC2)"
      mask Display:
      | disp('PSS2A')
      | 
      | port_label('input',1,'dw')
      | port_label('input',2,'Pg')
      | %port_label('input',3,'Vs')
      | 
      | port_label('output',1,'Vs')
  SEXS : Subsystem  mask{K=200, Ta=3, Tb=10, Te=0.05, Emin=-4, Emax=4, Vf0=1.16721}
      mask prompts: K "Controller gain (K)"; Ta "Filter derivative time constant (Ta)(sec)"; Tb "Filter delay time (Tb)(sec)"; Te "Exciter time constant (Te)(sec)"; Emin "Controller minimum output (Emin)"; Emax "Controller maximum output (Emax)"; Vf0 "Initial output (p.u)"
      mask Display:
      | disp('AVR')
      | 
      | port_label('input',1,'Vref')
      | port_label('input',2,'Vc')
      | port_label('input',3,'Vs')
      | 
      | port_label('output',1,'Efd')
  TR and LC_test : Subsystem  mask{Tr=1e-3, Rc=0, Xc=0}
      mask prompts: Tr "Transducter filter time constant (Tr)(sec)"; Rc "Resistance to compensate (p.u)"; Xc "Reactance to compensate (p.u)"
      mask Display:
      | %disp('Transducer \n \n')
      | %disp('and \n')
      | %disp('Load compensation')
      | text(15,35, 'Transducer')
      | text(30,24, 'and')
      | text(15,14, 'Load comp')
      | 
      | port_label('input',1,'Vt')
      | port_label('input',2,'It')
      | 
      | port_label('output',1,'Vc')
  Efd : Outport
  wires:
  TR and LC_test/1(Vc) -> SEXS/2(Vc)
  Vref/1 -> SEXS/1(Vref)
  Vt/1 -> TR and LC_test/1(Vt)
  <dw>/1 -> PSS1/1(dw)
  <Peo>/1 -> PSS1/2(Pgen)
  PSS1/1(Vothsg) -> SEXS/3(Vs)
  It/1 -> TR and LC_test/2(It)
  SEXS/1(Efd) -> Efd/1

== system SG_GFOL_2020a/G1/Speed Governor ==
  note: mechanical power
  RefL : Inport
  dw : Inport  Port=2
  Gain1 : Gain  Gain=Dt
  Gain2 : Gain  Gain=1/R
  Saturation : Saturate  UpperLimit=Vmax  LowerLimit=Vmin
  Saturation1 : Saturate  UpperLimit=1
  Sum : Sum  Inputs=|+-
  Sum1 : Sum  Inputs=|+-
  Transfer Fcn (with initial outputs)1 : simulink_extras/Additional Linear/Transfer Fcn (with initial outputs)  N=[T2 1]  D=[T3 1]  Y0=P0  U0=P0
  Transfer Fcn (with initial outputs)2 : simulink_extras/Additional Linear/Transfer Fcn (with initial outputs)  N=[1]  D=[T1 1]  Y0=P0  U0=P0
  Pm : Outport
  wires:
  Saturation1/1 -> Pm/1
  RefL/1 -> Sum/1
  Sum/1 -> Transfer Fcn (with initial outputs)2/1
  Transfer Fcn (with initial outputs)2/1 -> Saturation/1
  Saturation/1 -> Transfer Fcn (with initial outputs)1/1
  Sum1/1 -> Saturation1/1
  Transfer Fcn (with initial outputs)1/1 -> Sum1/1
  Gain1/1 -> Sum1/2
  dw/1 -> Gain1/1, Gain2/1
  Gain2/1 -> Sum/2

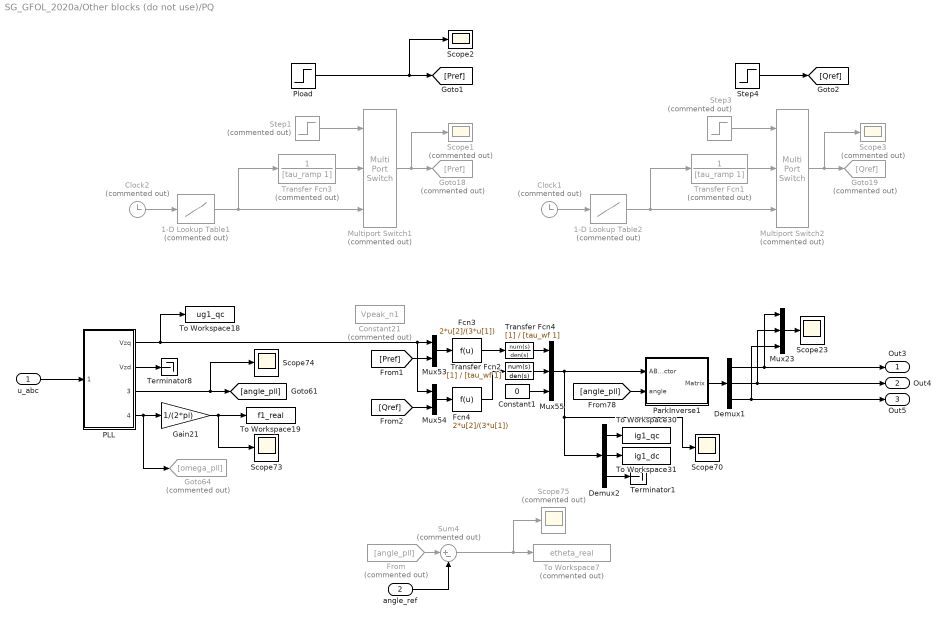
== system SG_GFOL_2020a/Other blocks (do not use)/PQ ==
  u_abc : Inport
  angle_ref : Inport  Port=2
  1-D Lookup Table1 : Lookup_n-D  Commented=on  NumberOfTableDimensions=1  BreakpointsForDimension1=[0,t_ramp,t_step_P]  Table=[0,P_set,P_step]  InterpMethod=Flat  InternalRulePriority=Speed  RndMeth=Simplest
  1-D Lookup Table2 : Lookup_n-D  Commented=on  NumberOfTableDimensions=1  BreakpointsForDimension1=[0,t_ramp,t_step_Q]  Table=[0,Q_set,Q_step]  InterpMethod=Flat  InternalRulePriority=Speed  RndMeth=Simplest
  Clock1 : Clock  Commented=on
  Clock2 : Clock  Commented=on
  Constant1 : Constant  Value=0
  Constant21 : Constant  Commented=on  Value=Vpeak_n1
  Demux1 : Demux  Outputs=3
  Demux2 : Demux  Outputs=3
  Fcn3 : Fcn  Expr=2*u[2]/(3*u[1])
  Fcn4 : Fcn  Expr=2*u[2]/(3*u[1])
  From : From  Commented=on  GotoTag=angle_pll
  Gain21 : Gain  Gain=1/(2*pi)
  Goto18 : Goto  Commented=on  GotoTag=Pref
  Goto19 : Goto  Commented=on  GotoTag=Qref
  Goto64 : Goto  Commented=on  GotoTag=omega_pll
  Multiport Switch1 : MultiPortSwitch  Commented=on  Inputs=2  SaturateOnIntegerOverflow=off  InputSameDT=off
  Multiport Switch2 : MultiPortSwitch  Commented=on  Inputs=2  SaturateOnIntegerOverflow=off  InputSameDT=off
  Mux23 : Mux  Inputs=3
  Mux53 : Mux  Inputs=2
  Mux54 : Mux  Inputs=2
  Mux55 : Mux  Inputs=3
  PLL : Subsystem
  ParkInverse1 : Subsystem  mask(Gerard){}
      mask help:
      | This block applies the park inverse transfomation from a desired vector.
      | The input Xqd0 refers to the vector in the qd0 frame, and the second input is the angle used in the inverse transformation.
      | The output is the vector in the ABC frame.
      mask Display:
      | port_label('output',1,'Xabc')
      | port_label('input',1,'Xqd0')
      | port_label('input',2,'angle')
  Pload : Step  Time=T_stp  Before=Pload_init  After=Pload_fnl  SampleTime=0
  Scope1 : Scope  Commented=on
  Scope{2,23,70,73..74} (5 alike) : Scope
  Scope3 : Scope  Commented=on
  Scope75 : Scope  Commented=on
  Step1 : Step  Commented=on  Time=t_step_P-0.01  Before=1  After=2  SampleTime=0
  Step3 : Step  Commented=on  Time=t_step_Q-0.01  Before=1  After=2  SampleTime=0
  Step4 : Step  After=0  SampleTime=0
  Sum4 : Sum  Commented=on  Inputs=|+-
  Terminator1 : Terminator
  Terminator8 : Terminator
  To Workspace18 : ToWorkspace  VariableName=ug1_qc  SampleTime=plots_step
  To Workspace19 : ToWorkspace  VariableName=f1_real  SampleTime=plots_step
  To Workspace30 : ToWorkspace  VariableName=ig1_qc  SampleTime=plots_step
  To Workspace31 : ToWorkspace  VariableName=ig1_dc  SampleTime=plots_step
  To Workspace7 : ToWorkspace  Commented=on  VariableName=etheta_real  SampleTime=plots_step
  Transfer Fcn1 : TransferFcn  Commented=on  Denominator=[tau_ramp 1]
  Transfer Fcn2 : TransferFcn  Denominator=[tau_wf 1]
  Transfer Fcn3 : TransferFcn  Commented=on  Denominator=[tau_ramp 1]
  Transfer Fcn4 : TransferFcn  Denominator=[tau_wf 1]
  Out3 : Outport
  Out4 : Outport  Port=2
  Out5 : Outport  Port=3
  wires:
  Fcn3/1 -> Transfer Fcn4/1
  Demux2/2 -> To Workspace31/1
  Demux1/3 -> Out5/1, Mux23/3
  Transfer Fcn2/1 -> Mux55/2
  Demux1/1 -> Out3/1, Mux23/1
  Transfer Fcn4/1 -> Mux55/1
  Demux1/2 -> Out4/1, Mux23/2
  Mux23/1 -> Scope23/1
  u_abc/1 -> PLL/1(u_abc)
  ParkInverse1/1(Matrix) -> Demux1/1
  [Pref] -> Mux53/2
  Mux55/1 -> ParkInverse1/1(ABC vector), Demux2/1, Scope70/1
  [Qref] -> Mux54/2
  Gain21/1 -> To Workspace19/1, Scope73/1
  PLL/4(w_grid) -> Goto64/1, Gain21/1
  Demux2/1 -> To Workspace30/1
  Mux54/1 -> Fcn4/1
  Fcn4/1 -> Transfer Fcn2/1
  angle_ref/1 -> Sum4/2
  PLL/3(angle) -> Scope74/1, [angle_pll]
  Mux53/1 -> Fcn3/1
  Sum4/1 -> To Workspace7/1, Scope75/1
  [angle_pll] -> ParkInverse1/2(angle)
  From/1 -> Sum4/1
  PLL/1(Vzq) -> To Workspace18/1, Mux54/1, Mux53/1
  PLL/2(Vzd) -> Terminator8/1
  Demux2/3 -> Terminator1/1
  Constant1/1 -> Mux55/3
  Clock1/1 -> 1-D Lookup Table2/1
  Multiport Switch1/1 -> Scope1/1, Goto18/1
  Transfer Fcn1/1 -> Multiport Switch2/2
  Clock2/1 -> 1-D Lookup Table1/1
  Multiport Switch2/1 -> Scope3/1, Goto19/1
  1-D Lookup Table2/1 -> Transfer Fcn1/1, Multiport Switch2/3
  Step1/1 -> Multiport Switch1/1
  Transfer Fcn3/1 -> Multiport Switch1/2
  1-D Lookup Table1/1 -> Multiport Switch1/3, Transfer Fcn3/1
  Step3/1 -> Multiport Switch2/1
  Pload/1 -> Scope2/1, [Pref]
  Step4/1 -> [Qref]

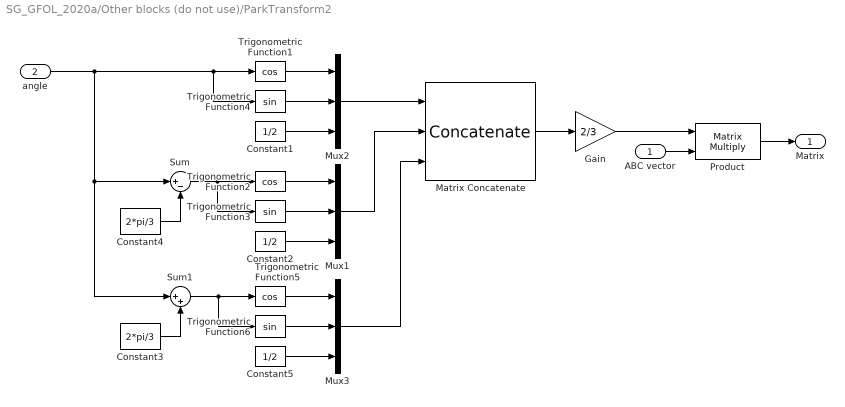
== system SG_GFOL_2020a/Other blocks (do not use)/ParkTransform2 ==
  ABC vector : Inport
  angle : Inport  Port=2
  Constant1 : Constant  Value=1/2
  Constant2 : Constant  Value=1/2
  Constant3 : Constant  Value=2*pi/3
  Constant4 : Constant  Value=2*pi/3
  Constant5 : Constant  Value=1/2
  Gain : Gain  Gain=2/3
  Matrix Concatenate : Concatenate  NumInputs=3  Mode=Multidimensional array  ConcatenateDimension=2
  Mux1 : Mux  Inputs=3
  Mux2 : Mux  Inputs=3
  Mux3 : Mux  Inputs=3
  Product : Product  Multiplication=Matrix(*)  RndMeth=Zero
  Sum : Sum  Inputs=|+-
  Sum1 : Sum  Inputs=|++
  Trigonometric Function1 : Trigonometry  Operator=cos
  Trigonometric Function2 : Trigonometry  Operator=cos
  Trigonometric Function3 : Trigonometry
  Trigonometric Function4 : Trigonometry
  Trigonometric Function5 : Trigonometry  Operator=cos
  Trigonometric Function6 : Trigonometry
  Matrix : Outport
  wires:
  Matrix Concatenate/1 -> Gain/1
  ABC vector/1 -> Product/2
  Product/1 -> Matrix/1
  Gain/1 -> Product/1
  Constant4/1 -> Sum/2
  Constant3/1 -> Sum1/2
  angle/1 -> Trigonometric Function4/1, Trigonometric Function1/1, Sum1/1, Sum/1
  Trigonometric Function3/1 -> Mux1/2
  Trigonometric Function2/1 -> Mux1/1
  Constant2/1 -> Mux1/3
  Sum/1 -> Trigonometric Function3/1, Trigonometric Function2/1
  Trigonometric Function4/1 -> Mux2/2
  Trigonometric Function1/1 -> Mux2/1
  Constant1/1 -> Mux2/3
  Trigonometric Function6/1 -> Mux3/2
  Trigonometric Function5/1 -> Mux3/1
  Constant5/1 -> Mux3/3
  Sum1/1 -> Trigonometric Function6/1, Trigonometric Function5/1
  Mux1/1 -> Matrix Concatenate/2
  Mux2/1 -> Matrix Concatenate/1
  Mux3/1 -> Matrix Concatenate/3

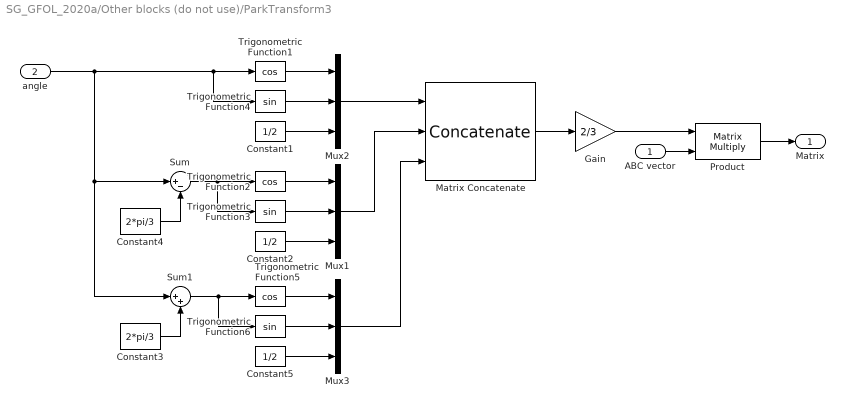
== system SG_GFOL_2020a/Other blocks (do not use)/ParkTransform3 ==
  ABC vector : Inport
  angle : Inport  Port=2
  Constant1 : Constant  Value=1/2
  Constant2 : Constant  Value=1/2
  Constant3 : Constant  Value=2*pi/3
  Constant4 : Constant  Value=2*pi/3
  Constant5 : Constant  Value=1/2
  Gain : Gain  Gain=2/3
  Matrix Concatenate : Concatenate  NumInputs=3  Mode=Multidimensional array  ConcatenateDimension=2
  Mux1 : Mux  Inputs=3
  Mux2 : Mux  Inputs=3
  Mux3 : Mux  Inputs=3
  Product : Product  Multiplication=Matrix(*)  RndMeth=Zero
  Sum : Sum  Inputs=|+-
  Sum1 : Sum  Inputs=|++
  Trigonometric Function1 : Trigonometry  Operator=cos
  Trigonometric Function2 : Trigonometry  Operator=cos
  Trigonometric Function3 : Trigonometry
  Trigonometric Function4 : Trigonometry
  Trigonometric Function5 : Trigonometry  Operator=cos
  Trigonometric Function6 : Trigonometry
  Matrix : Outport
  wires:
  Mux3/1 -> Matrix Concatenate/3
  Mux2/1 -> Matrix Concatenate/1
  Mux1/1 -> Matrix Concatenate/2
  Sum1/1 -> Trigonometric Function5/1, Trigonometric Function6/1
  Constant5/1 -> Mux3/3
  Trigonometric Function5/1 -> Mux3/1
  Trigonometric Function6/1 -> Mux3/2
  Constant1/1 -> Mux2/3
  Trigonometric Function1/1 -> Mux2/1
  Trigonometric Function4/1 -> Mux2/2
  Sum/1 -> Trigonometric Function2/1, Trigonometric Function3/1
  Constant2/1 -> Mux1/3
  Trigonometric Function2/1 -> Mux1/1
  Trigonometric Function3/1 -> Mux1/2
  angle/1 -> Sum/1, Sum1/1, Trigonometric Function1/1, Trigonometric Function4/1
  Constant3/1 -> Sum1/2
  Constant4/1 -> Sum/2
  Gain/1 -> Product/1
  Product/1 -> Matrix/1
  ABC vector/1 -> Product/2
  Matrix Concatenate/1 -> Gain/1

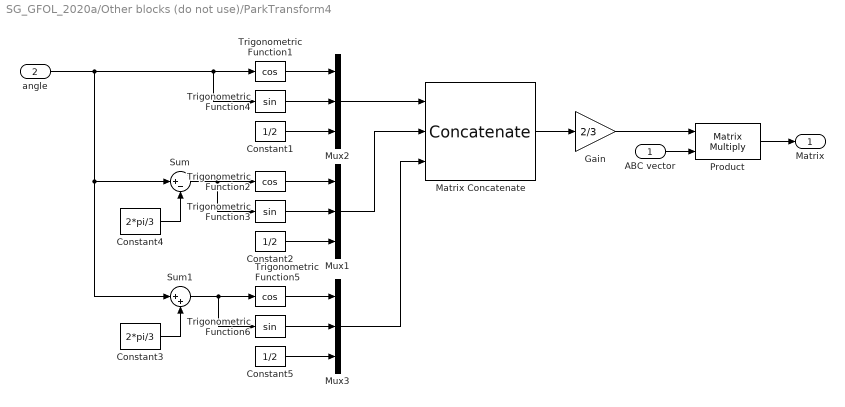
== system SG_GFOL_2020a/Other blocks (do not use)/ParkTransform4 ==
  ABC vector : Inport
  angle : Inport  Port=2
  Constant1 : Constant  Value=1/2
  Constant2 : Constant  Value=1/2
  Constant3 : Constant  Value=2*pi/3
  Constant4 : Constant  Value=2*pi/3
  Constant5 : Constant  Value=1/2
  Gain : Gain  Gain=2/3
  Matrix Concatenate : Concatenate  NumInputs=3  Mode=Multidimensional array  ConcatenateDimension=2
  Mux1 : Mux  Inputs=3
  Mux2 : Mux  Inputs=3
  Mux3 : Mux  Inputs=3
  Product : Product  Multiplication=Matrix(*)  RndMeth=Zero
  Sum : Sum  Inputs=|+-
  Sum1 : Sum  Inputs=|++
  Trigonometric Function1 : Trigonometry  Operator=cos
  Trigonometric Function2 : Trigonometry  Operator=cos
  Trigonometric Function3 : Trigonometry
  Trigonometric Function4 : Trigonometry
  Trigonometric Function5 : Trigonometry  Operator=cos
  Trigonometric Function6 : Trigonometry
  Matrix : Outport
  wires:
  Mux3/1 -> Matrix Concatenate/3
  Mux2/1 -> Matrix Concatenate/1
  Mux1/1 -> Matrix Concatenate/2
  Sum1/1 -> Trigonometric Function5/1, Trigonometric Function6/1
  Constant5/1 -> Mux3/3
  Trigonometric Function5/1 -> Mux3/1
  Trigonometric Function6/1 -> Mux3/2
  Constant1/1 -> Mux2/3
  Trigonometric Function1/1 -> Mux2/1
  Trigonometric Function4/1 -> Mux2/2
  Sum/1 -> Trigonometric Function2/1, Trigonometric Function3/1
  Constant2/1 -> Mux1/3
  Trigonometric Function2/1 -> Mux1/1
  Trigonometric Function3/1 -> Mux1/2
  angle/1 -> Sum/1, Sum1/1, Trigonometric Function1/1, Trigonometric Function4/1
  Constant3/1 -> Sum1/2
  Constant4/1 -> Sum/2
  Gain/1 -> Product/1
  Product/1 -> Matrix/1
  ABC vector/1 -> Product/2
  Matrix Concatenate/1 -> Gain/1

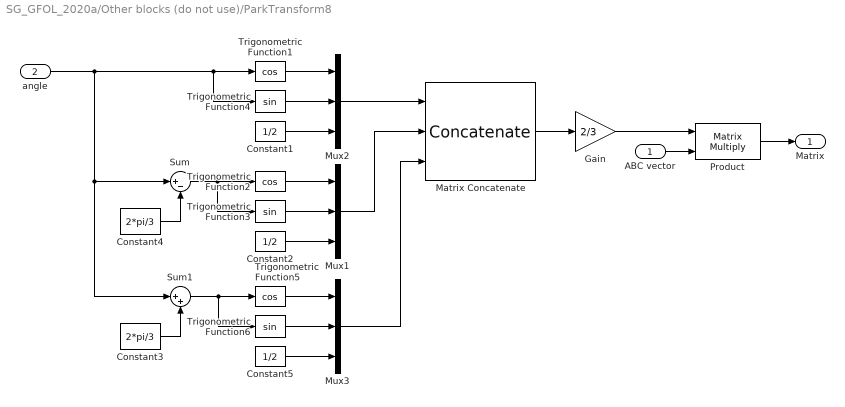
== system SG_GFOL_2020a/Other blocks (do not use)/ParkTransform8 ==
  ABC vector : Inport
  angle : Inport  Port=2
  Constant1 : Constant  Value=1/2
  Constant2 : Constant  Value=1/2
  Constant3 : Constant  Value=2*pi/3
  Constant4 : Constant  Value=2*pi/3
  Constant5 : Constant  Value=1/2
  Gain : Gain  Gain=2/3
  Matrix Concatenate : Concatenate  NumInputs=3  Mode=Multidimensional array  ConcatenateDimension=2
  Mux1 : Mux  Inputs=3
  Mux2 : Mux  Inputs=3
  Mux3 : Mux  Inputs=3
  Product : Product  Multiplication=Matrix(*)  RndMeth=Zero
  Sum : Sum  Inputs=|+-
  Sum1 : Sum  Inputs=|++
  Trigonometric Function1 : Trigonometry  Operator=cos
  Trigonometric Function2 : Trigonometry  Operator=cos
  Trigonometric Function3 : Trigonometry
  Trigonometric Function4 : Trigonometry
  Trigonometric Function5 : Trigonometry  Operator=cos
  Trigonometric Function6 : Trigonometry
  Matrix : Outport
  wires:
  Matrix Concatenate/1 -> Gain/1
  ABC vector/1 -> Product/2
  Product/1 -> Matrix/1
  Gain/1 -> Product/1
  Constant4/1 -> Sum/2
  Constant3/1 -> Sum1/2
  angle/1 -> Trigonometric Function4/1, Trigonometric Function1/1, Sum1/1, Sum/1
  Trigonometric Function3/1 -> Mux1/2
  Trigonometric Function2/1 -> Mux1/1
  Constant2/1 -> Mux1/3
  Sum/1 -> Trigonometric Function3/1, Trigonometric Function2/1
  Trigonometric Function4/1 -> Mux2/2
  Trigonometric Function1/1 -> Mux2/1
  Constant1/1 -> Mux2/3
  Trigonometric Function6/1 -> Mux3/2
  Trigonometric Function5/1 -> Mux3/1
  Constant5/1 -> Mux3/3
  Sum1/1 -> Trigonometric Function6/1, Trigonometric Function5/1
  Mux1/1 -> Matrix Concatenate/2
  Mux2/1 -> Matrix Concatenate/1
  Mux3/1 -> Matrix Concatenate/3
